simulink model "VCU_TDN"  (R2020a)
settings: Solver=FixedStepDiscrete  StartTime=0.0  StopTime=10.0  FixedStep=0.001  RelTol=1e-3  EnableMultiTasking=on
InitFcn:
  | EcoCoder_PreCheckLic();
undefined symbols (not defined in the file or in its folder): h, km
libraries: CoderSF_BSW_Libs x187, simulink x9, SF_CanService_Libs x1
(part 1 of 2)
settings Model: Creator=timot  LastModifiedBy=Thibault NOUVELLON
settings DataIOCC: SaveFormat=Structure  SignalLoggingSaveFormat=ModelDataLogs  SaveOutput=off  SignalLogging=off  DSMLogging=off  SaveTime=off  ReturnWorkspaceOutputs=off
settings OptimizationCC: DefaultParameterBehavior=Inlined  InlineInvariantSignals=on  EnhancedBackFolding=on  StrengthReduction=on  EnableMemcpy=off  PassReuseOutputArgsAs=Individual arguments  EfficientFloat2IntCast=on  LifeSpan=1  SimCompilerOptimization=on  OptimizeBlockOrder=speed  DifferentSizesBufferReuse=on  EfficientTunableParamExpr=on
settings DebuggingCC: AlgebraicLoopMsg=none  ArtificialAlgebraicLoopMsg=none  SaveWithDisabledLinksMsg=none  SaveWithParameterizedLinksMsg=none  CheckSSInitialOutputMsg=off  UnderspecifiedInitializationDetection=Classic  SignalResolutionControl=TryResolveAll  BlockPriorityViolationMsg=error  MinStepSizeMsg=none  InheritedTsInSrcMsg=none  MultiTaskDSMMsg=none  MultiTaskCondExecSysMsg=none  MultiTaskRateTransMsg=warning  TasksWithSamePriorityMsg=none  SigSpecEnsureSampleTimeMsg=none  IntegerOverflowMsg=error  Int32ToFloatConvMsg=none  ParameterPrecisionLossMsg=none  ParameterTunabilityLossMsg=none  FixptConstOverflowMsg=error  FcnCallInpInsideContextMsg=warning  UnconnectedInputMsg=error  UnconnectedOutputMsg=error  UnconnectedLineMsg=error  FrameProcessingCompatibilityMsg=none  BusObjectLabelMismatch=none  RootOutportRequireBusObject=none  UnknownTsInhSupMsg=none  ModelReferenceDataLoggingMessage=none  OperatingPointInterfaceChecksumMismatchMsg=none  SFUnusedDataAndEventsDiag=none  SFUnexpectedBacktrackingDiag=none  SFInvalidInputDataAccessInChartInitDiag=none  SFNoUnconditionalDefaultTransitionDiag=none  SFTransitionOutsideNaturalParentDiag=none  SFUnreachableExecutionPathDiag=none  SFMachineParentedDataDiag=error
settings HardwareCC: ProdBitPerPointer=32  ProdBitPerSizeT=32  ProdBitPerPtrDiffT=32  ProdLargestAtomicInteger=Long  ProdLargestAtomicFloat=Double  ProdEndianess=BigEndian  ProdWordSize=32  ProdHWDeviceType=Freescale->MPC55xx
settings ModelReferenceCC: UpdateModelReferenceTargets=Force  ModelReferenceNumInstancesAllowed=Single  PropagateSignalLabelsOutOfModel=off
settings SFSimCC: SFSimEcho=off  MATLABDynamicMemAlloc=off
settings RTWCC: Description=Ecotrons MPC5xxx  SystemTargetFile=MPC5644A.tlc  GenerateMakefile=off  TemplateMakefile=ert_default_tmf  RTWVerbose=off  RetainRTWFile=on  RTWCompilerOptimization=on
settings CodeAppCC: IgnoreCustomStorageClasses=off  OperatorAnnotations=on  CustomSymbolStrGlobalVar=$N$M  CustomSymbolStrType=$N$M  CustomSymbolStrFcn=$N$M  CustomSymbolStrFcnArg=$N$M  CustomSymbolStrBlkIO=$N$M  CustomSymbolStrMacro=$N$M
settings STFCustomTargetCC: UtilityFuncGeneration=Shared location  MultiwordLength=256  IncludeMdlTerminateFcn=off  CombineOutputUpdateFcns=on  SuppressErrorStatus=on  ERTCustomFileBanners=on  SupportNonFinite=off  SupportComplex=off  SupportContinuousTime=off  SupportNonInlinedSFcns=off  MATLABClassNameForMDSCustomization=Simulink.SoftwareTarget.ERTCustomization  SystemTargetFile=MPC5644A.tlc
settings ERTTargetCC: UtilityFuncGeneration=Shared location  ParMdlRefBuildCompliant=off  CompOptLevelCompliant=off  ConcurrentExecutionCompliant=off  IncludeMdlTerminateFcn=off  SuppressErrorStatus=on  SupportNonFinite=off  SupportComplex=off  RemoveResetFunc=off  ModelStepFunctionPrototypeControlCompliant=off  CPPClassGenCompliant=off  UseToolchainInfoCompliant=off  GenerateASAP2=on  InlinedParameterPlacement=NonHierarchical  ERTCustomFileTemplate=MPC5644A_file_process.tlc  ERTFilePackagingFormat=Compact  PreserveIfCondition=on  ConvertIfToSwitch=off  PreserveExternInFcnDecls=off  SuppressUnreachableDefaultCases=off

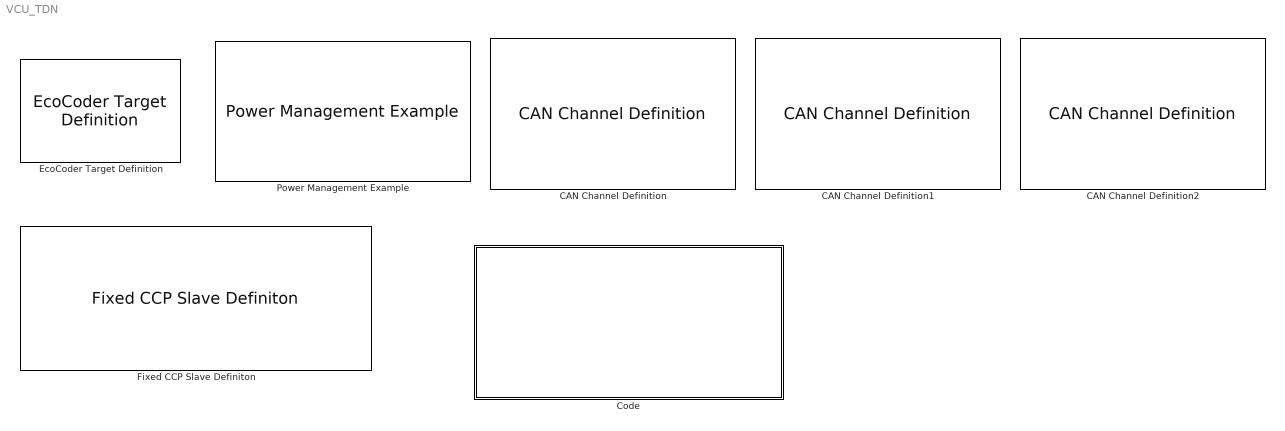
== system VCU_TDN ==
  CAN Channel Definition : CoderSF_BSW_Libs/CAN/CAN Channel Definition  Priority=2  channel=CAN_A  can_en=on  can_idfilter=off  can_rxextended=off  can_rxMask=hex2dec('7ff')  can_rxID=hex2dec('100')  can_baudrateIndex=500  can_txbuffer_size=30  can_rxbuffer_size=1  can_en_fd=off  nominalSamplePoint=7500  can_baudrateIndex_data=500  fastSamplePoint=7500  canfd_txbuffer_size=5  EcoCoderBlockID=C001_CANDef
  CAN Channel Definition1 : CoderSF_BSW_Libs/CAN/CAN Channel Definition  Priority=3  channel=CAN_B  can_en=on  can_idfilter=off  can_rxextended=off  can_rxMask=hex2dec('7ff')  can_rxID=hex2dec('100')  can_baudrateIndex=500  can_txbuffer_size=30  can_rxbuffer_size=1  can_en_fd=off  nominalSamplePoint=7500  can_baudrateIndex_data=500  fastSamplePoint=7500  canfd_txbuffer_size=5  EcoCoderBlockID=C001_CANDef
  CAN Channel Definition2 : CoderSF_BSW_Libs/CAN/CAN Channel Definition  Priority=4  channel=CAN_C  can_en=on  can_idfilter=off  can_rxextended=off  can_rxMask=hex2dec('7ff')  can_rxID=hex2dec('100')  can_baudrateIndex=500  can_txbuffer_size=30  can_rxbuffer_size=1  can_en_fd=off  nominalSamplePoint=7500  can_baudrateIndex_data=500  fastSamplePoint=7500  canfd_txbuffer_size=5  EcoCoderBlockID=C001_CANDef
  Code : Subsystem  Priority=6
  EcoCoder Target Definition : CoderSF_BSW_Libs/EcoCoder Target Definition  targetECU=EV2274A  EcoCoderBlockID=T001_Target  enNoTriggerCall=on  flgBlockReduction=on  flgShowDebugDisp=off  flgDisTargetOutFIleCounter=off  flgClearAllOldFiles=on  tc275_cal_len=hex2dec('00008000')  internal_flash=[hex2dec('00020000'),hex2dec('000E0000')]  cal_rom_phy=[hex2dec('00010000'),hex2dec('00002000')]  cal_ram_wp=[hex2dec('4000F000'),hex2dec('00002000')]  cal_ram_msm=[hex2dec('40000000'),hex2dec('00002000')]  var_ram_wp=[hex2dec('40002000'),hex2dec('0000D000')]  write_back_fixed_ram=[hex2dec('40011000'),hex2dec('00001000')]  write_back_unfixed_ram=[hex2dec('40012000'),hex2dec('00001000')]  stack=[hex2dec('40013000'),hex2dec('00001000')]
      settings: AttributesFormatString=Target :%<targetECU>
  Fixed CCP Slave Definiton : CoderSF_BSW_Libs/CCP/Fixed CCP Slave Definiton  Priority=5  ccpType=Configurable  ccp_enSet=on  ccp_disASW=on  channel=CAN_B  stationaddressSet=hex2dec('0112')  croidSet=hex2dec('100')  dtoidSet=hex2dec('101')  daqidSet=[hex2dec('101') hex2dec('101') hex2dec('101') hex2dec('102')]  daqpidSet=[hex2dec('0') hex2dec('3C') hex2dec('78') hex2dec('0')]  daqlenSet=[hex2dec('0') hex2dec('20') hex2dec('30') hex2dec('30')]  daqperSet=[5 20 100 0]  EcoCoderBlockID=C002_CCP21Conf
  Power Management Example : CoderSF_BSW_Libs/System Management Blocks/Power Management Example  Priority=1  flgKeyFromIn=off  tKeyOffDelaySet=0.5  flgResetSWEnSet=1  tDbncKeyOffFallSet=0.1  tDbncKeyOffRiseSet=0.1  facAd2VoltSet=109/27846  uKeyOffThrSet=1  uKeyOnHystSet=1  flgCANRxLiveCheckEn=0  flgEnPwrDwnFailReset=0  flgNVMEn=on  tShtDwnWait=500  flgPwrDwnByEdgeTrigger=off  EcoCoderBlockID=PME001_Def
      settings: AttributesFormatString=Priority:%<Priority>

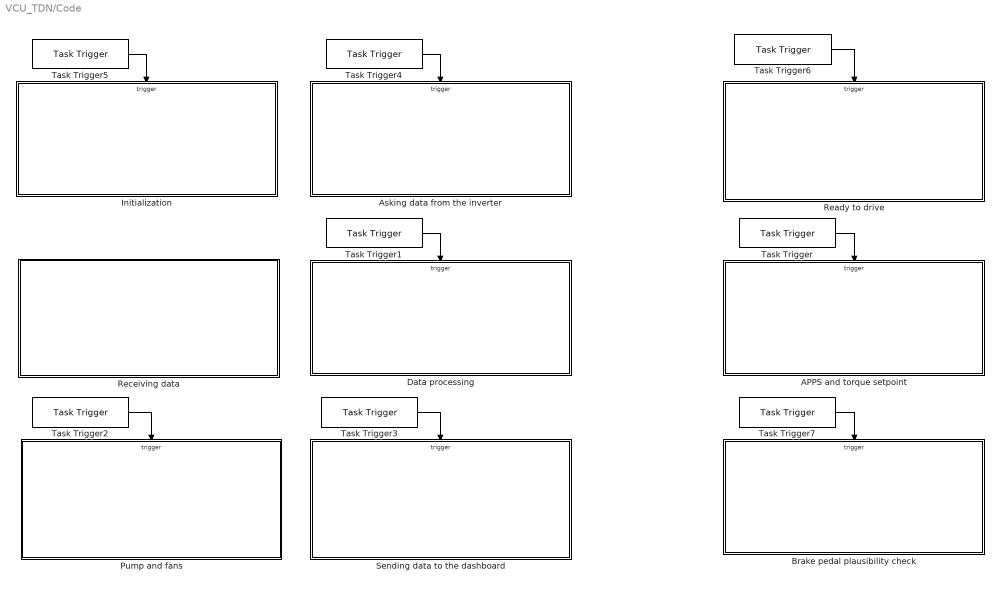
== system VCU_TDN/Code ==
  APPS and torque setpoint : Subsystem
  Asking data from the inverter : Subsystem
  Brake pedal plausibility check : Subsystem
  Data processing : Subsystem
  Initialization : Subsystem
  Pump and fans : Subsystem
  Ready to drive : Subsystem
  Receiving data : Subsystem
  Sending data to the dashboard : Subsystem
  Task Trigger : CoderSF_BSW_Libs/Task Scheduler/Task Trigger  Priority=1  tasktimeIndex=Task_H1ms  PrioritySet=1
  Task Trigger1 : CoderSF_BSW_Libs/Task Scheduler/Task Trigger  Priority=1  tasktimeIndex=Task_L100ms  PrioritySet=1
  Task Trigger2 : CoderSF_BSW_Libs/Task Scheduler/Task Trigger  Priority=1  tasktimeIndex=Task_L1000ms  PrioritySet=1
  Task Trigger3 : CoderSF_BSW_Libs/Task Scheduler/Task Trigger  Priority=2  tasktimeIndex=Task_L100ms  PrioritySet=2
  Task Trigger4 : CoderSF_BSW_Libs/Task Scheduler/Task Trigger  Priority=2  tasktimeIndex=Task_ini  PrioritySet=2
  Task Trigger5 : CoderSF_BSW_Libs/Task Scheduler/Task Trigger  Priority=1  tasktimeIndex=Task_ini  PrioritySet=1
  Task Trigger6 : CoderSF_BSW_Libs/Task Scheduler/Task Trigger  Priority=3  tasktimeIndex=Task_H1ms  PrioritySet=3
  Task Trigger7 : CoderSF_BSW_Libs/Task Scheduler/Task Trigger  Priority=2  tasktimeIndex=Task_H1ms  PrioritySet=2
  wires:
  Task Trigger/1 -> APPS and torque setpoint/Trigger
  Task Trigger3/1 -> Sending data to the dashboard/Trigger
  Task Trigger4/1 -> Asking data from the inverter/Trigger
  Task Trigger1/1 -> Data processing/Trigger
  Task Trigger2/1 -> Pump and fans/Trigger
  Task Trigger5/1 -> Initialization/Trigger
  Task Trigger6/1 -> Ready to drive/Trigger
  Task Trigger7/1 -> Brake pedal plausibility check/Trigger

== system VCU_TDN/Code/APPS and torque setpoint ==
  Trigger : TriggerPort  TriggerType=function-call  VariantControl=Variant  PortDimensions=1
  APPS 1 : CoderSF_BSW_Libs/ADC/Read ADC Value  channel=6
  APPS 2 : CoderSF_BSW_Libs/ADC/Read ADC Value  channel=7
  APPS Fault detection : Subsystem
  Throttle setpoint for the inverter : Subsystem
  Write NVM : CoderSF_BSW_Libs/Non-volatile Memory Blocks/Write NVM  variable_name=nvmAPPS_1  flgDef=on  variable_value=0  variable_type=uint16  variable_numD=1  unitStr=""  descStr=""  EcoCoderBlockID=N001_NVMVDEF
      settings: AttributesFormatString=value:%<variable_value> type:%<variable_type> D:%<variable_numD>
  Write NVM1 : CoderSF_BSW_Libs/Non-volatile Memory Blocks/Write NVM  variable_name=nvmAPPS_2  flgDef=on  variable_value=0  variable_type=uint16  variable_numD=1  unitStr=""  descStr=""  EcoCoderBlockID=N001_NVMVDEF
      settings: AttributesFormatString=value:%<variable_value> type:%<variable_type> D:%<variable_numD>
  Write and Read Measurement : CoderSF_BSW_Libs/Calibration & Measurement/Write and Read Measurement  variable_name=APPS_1  variable_value=0  variable_type=uint16  numD=1  unitStr=""  descStr=""
      settings: AttributesFormatString=type:%<variable_type> Dimensions:%<numD>
  Write and Read Measurement1 : CoderSF_BSW_Libs/Calibration & Measurement/Write and Read Measurement  variable_name=APPS_2  variable_value=0  variable_type=uint16  numD=1  unitStr=""  descStr=""
      settings: AttributesFormatString=type:%<variable_type> Dimensions:%<numD>
  wires:
  APPS 1/1 -> Write NVM/1, Write and Read Measurement/1
  Write and Read Measurement/1 -> Throttle setpoint for the inverter/1(APPS 1), APPS Fault detection/1(APPS 1)  "APPS_1"
  APPS 2/1 -> Write NVM1/1, Write and Read Measurement1/1
  Write and Read Measurement1/1 -> Throttle setpoint for the inverter/2(APPS 2), APPS Fault detection/2(APPS 2)  "APPS_2"

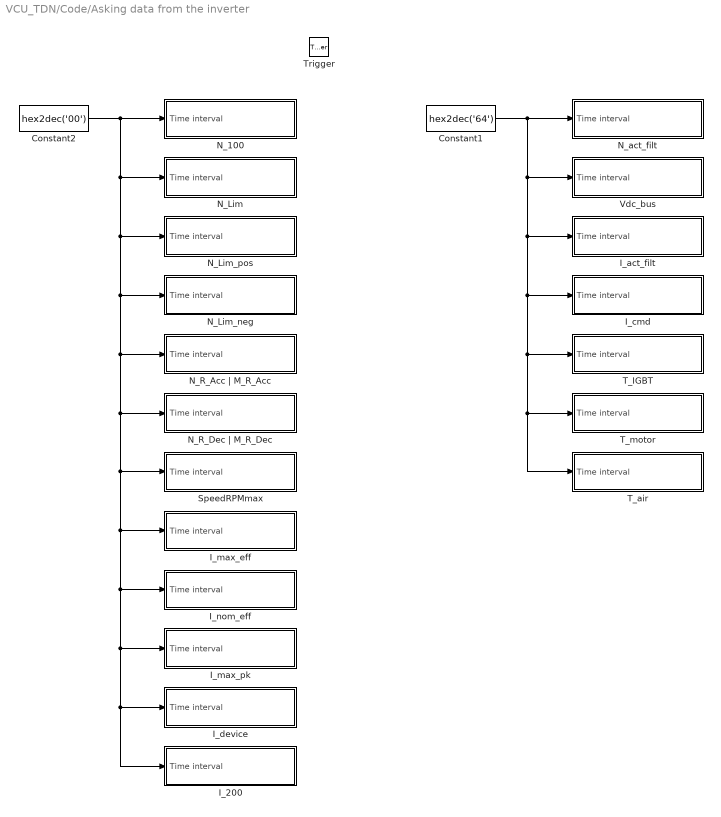
== system VCU_TDN/Code/Asking data from the inverter ==
  Trigger : TriggerPort  TriggerType=function-call  VariantControl=Variant  PortDimensions=1
  Constant1 : Constant  Value=hex2dec('64')  OutDataTypeStr=uint8
  Constant2 : Constant  Value=hex2dec('00')  OutDataTypeStr=uint8
  I_200 : Subsystem
  I_act_filt : Subsystem
  I_cmd : Subsystem
  I_device : Subsystem
  I_max_eff : Subsystem
  I_max_pk : Subsystem
  I_nom_eff : Subsystem
  N_100 : Subsystem
  N_Lim : Subsystem
  N_Lim_neg : Subsystem
  N_Lim_pos : Subsystem
  N_R_Acc | M_R_Acc : Subsystem
  N_R_Dec | M_R_Dec : Subsystem
  N_act_filt : Subsystem
  SpeedRPMmax : Subsystem
  T_IGBT : Subsystem
  T_air : Subsystem
  T_motor : Subsystem
  Vdc_bus : Subsystem
  wires:
  Constant2/1 -> SpeedRPMmax/1(Time interval), I_200/1(Time interval), I_device/1(Time interval), I_max_pk/1(Time interval), I_nom_eff/1(Time interval), I_max_eff/1(Time interval), N_R_Dec | M_R_Dec/1(Time interval), N_R_Acc | M_R_Acc/1(Time interval), N_Lim_neg/1(Time interval), N_Lim_pos/1(Time interval), N_Lim/1(Time interval), N_100/1(Time interval)
  Constant1/1 -> T_air/1(Time interval), T_motor/1(Time interval), T_IGBT/1(Time interval), I_cmd/1(Time interval), I_act_filt/1(Time interval), Vdc_bus/1(Time interval), N_act_filt/1(Time interval)

== system VCU_TDN/Code/Brake pedal plausibility check ==
  Trigger : TriggerPort  TriggerType=function-call  VariantControl=Variant  PortDimensions=1
  Compare To Constant : simulink/Logic and Bit Operations/Compare To Constant  relop=>=  const=5  OutDataTypeStr=boolean
  Logical Operator : Logic  AllPortsSameDT=off  OutDataTypeStr=boolean
  Logical Operator1 : Logic  Inputs=1  AllPortsSameDT=off  OutDataTypeStr=boolean
  Read NVM : CoderSF_BSW_Libs/Non-volatile Memory Blocks/Read NVM  variable_name=nvmAPPS_M  variable_type=Inherit from 'Variable definition'
  Read NVM1 : CoderSF_BSW_Libs/Non-volatile Memory Blocks/Read NVM  variable_name=nvmBRK_CONTACTOR  variable_type=Inherit from 'Variable definition'
  Tapped Delay : simulink/Discrete/Tapped Delay  vinit=0.0  samptime=-1  NumDelays=490  DelayOrder=Oldest  includeCurrent=off
  Write Measurement : CoderSF_BSW_Libs/Calibration & Measurement/Write Measurement  variable_name=BRK_PDL_FAULT  variable_value=0  variable_type=boolean  numD=1  unitStr=""  descStr=""
      settings: AttributesFormatString=type:%<variable_type> Dimensions:%<numD>
  Write NVM : CoderSF_BSW_Libs/Non-volatile Memory Blocks/Write NVM  variable_name=nvmBRK_PDL_FAULT  flgDef=on  variable_value=0  variable_type=boolean  variable_numD=1  unitStr=""  descStr=""  EcoCoderBlockID=N001_NVMVDEF
      settings: AttributesFormatString=value:%<variable_value> type:%<variable_type> D:%<variable_numD>
  wires:
  Read NVM1/1 -> Logical Operator/2
  Logical Operator/1 -> Tapped Delay/1
  Tapped Delay/1 -> Logical Operator1/1
  Read NVM/1 -> Compare To Constant/1
  Compare To Constant/1 -> Logical Operator/1
  Logical Operator1/1 -> Write NVM/1, Write Measurement/1

== system VCU_TDN/Code/Data processing ==
  Trigger : TriggerPort  TriggerType=function-call  VariantControl=Variant  PortDimensions=1
  Electrical : Subsystem
  Speed : Subsystem
  Temperature : Subsystem

== system VCU_TDN/Code/Initialization ==
  Trigger : TriggerPort  TriggerType=function-call  VariantControl=Variant  PortDimensions=1
  Constant : Constant  Value=0  OutDataTypeStr=boolean
  Constant1 : Constant  Value=0  OutDataTypeStr=boolean
  Disabling the inverter : Subsystem
  FRG/RUN : CoderSF_BSW_Libs/Digital I//O/Switch Output  channel=LSO07
  NVM Definition : CoderSF_BSW_Libs/Non-volatile Memory Blocks/NVM Definition  load=Restore from factory default values in .mot  EcoCoderBlockID=N001_NVMDef
  RFE : CoderSF_BSW_Libs/Digital I//O/Switch Output  channel=LSO06
  wires:
  Constant/1 -> RFE/1
  Constant1/1 -> FRG/RUN/1

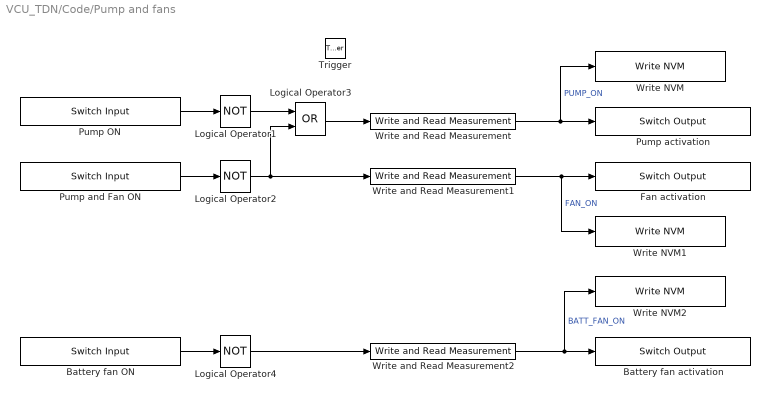
== system VCU_TDN/Code/Pump and fans ==
  Trigger : TriggerPort  TriggerType=function-call  VariantControl=Variant  PortDimensions=1
  Battery fan ON : CoderSF_BSW_Libs/Digital I//O/Switch Input  portNum=DI09
  Battery fan activation : CoderSF_BSW_Libs/Digital I//O/Switch Output  channel=LSO03
  Fan activation : CoderSF_BSW_Libs/Digital I//O/Switch Output  channel=LSO13
  Logical Operator1 : Logic  Operator=NOT  AllPortsSameDT=off  OutDataTypeStr=boolean
  Logical Operator2 : Logic  Operator=NOT  AllPortsSameDT=off  OutDataTypeStr=boolean
  Logical Operator3 : Logic  Operator=OR  AllPortsSameDT=off  OutDataTypeStr=boolean
  Logical Operator4 : Logic  Operator=NOT  AllPortsSameDT=off  OutDataTypeStr=boolean
  Pump ON : CoderSF_BSW_Libs/Digital I//O/Switch Input  portNum=DI12
  Pump activation : CoderSF_BSW_Libs/Digital I//O/Switch Output  channel=LSO12
  Pump and Fan ON : CoderSF_BSW_Libs/Digital I//O/Switch Input  portNum=DI12
  Write NVM : CoderSF_BSW_Libs/Non-volatile Memory Blocks/Write NVM  variable_name=nvmPUMP_ON  flgDef=on  variable_value=0  variable_type=boolean  variable_numD=1  unitStr=""  descStr=""  EcoCoderBlockID=N001_NVMVDEF
      settings: AttributesFormatString=value:%<variable_value> type:%<variable_type> D:%<variable_numD>
  Write NVM1 : CoderSF_BSW_Libs/Non-volatile Memory Blocks/Write NVM  variable_name=nvmFAN_ON  flgDef=on  variable_value=0  variable_type=boolean  variable_numD=1  unitStr=""  descStr=""  EcoCoderBlockID=N001_NVMVDEF
      settings: AttributesFormatString=value:%<variable_value> type:%<variable_type> D:%<variable_numD>
  Write NVM2 : CoderSF_BSW_Libs/Non-volatile Memory Blocks/Write NVM  variable_name=nvmBATT_FAN_ON  flgDef=on  variable_value=0  variable_type=boolean  variable_numD=1  unitStr=""  descStr=""  EcoCoderBlockID=N001_NVMVDEF
      settings: AttributesFormatString=value:%<variable_value> type:%<variable_type> D:%<variable_numD>
  Write and Read Measurement : CoderSF_BSW_Libs/Calibration & Measurement/Write and Read Measurement  variable_name=PUMP_ON  variable_value=0  variable_type=boolean  numD=1  unitStr=""  descStr=""
      settings: AttributesFormatString=type:%<variable_type> Dimensions:%<numD>
  Write and Read Measurement1 : CoderSF_BSW_Libs/Calibration & Measurement/Write and Read Measurement  variable_name=FAN_ON  variable_value=0  variable_type=boolean  numD=1  unitStr=""  descStr=""
      settings: AttributesFormatString=type:%<variable_type> Dimensions:%<numD>
  Write and Read Measurement2 : CoderSF_BSW_Libs/Calibration & Measurement/Write and Read Measurement  variable_name=BATT_FAN_ON  variable_value=0  variable_type=boolean  numD=1  unitStr=""  descStr=""
      settings: AttributesFormatString=type:%<variable_type> Dimensions:%<numD>
  wires:
  Logical Operator2/1 -> Write and Read Measurement1/1, Logical Operator3/2
  Pump and Fan ON/1 -> Logical Operator2/1
  Logical Operator1/1 -> Logical Operator3/1
  Logical Operator4/1 -> Write and Read Measurement2/1
  Logical Operator3/1 -> Write and Read Measurement/1
  Battery fan ON/1 -> Logical Operator4/1
  Pump ON/1 -> Logical Operator1/1
  Write and Read Measurement2/1 -> Write NVM2/1, Battery fan activation/1  "BATT_FAN_ON"
  Write and Read Measurement1/1 -> Write NVM1/1, Fan activation/1  "FAN_ON"
  Write and Read Measurement/1 -> Write NVM/1, Pump activation/1  "PUMP_ON"

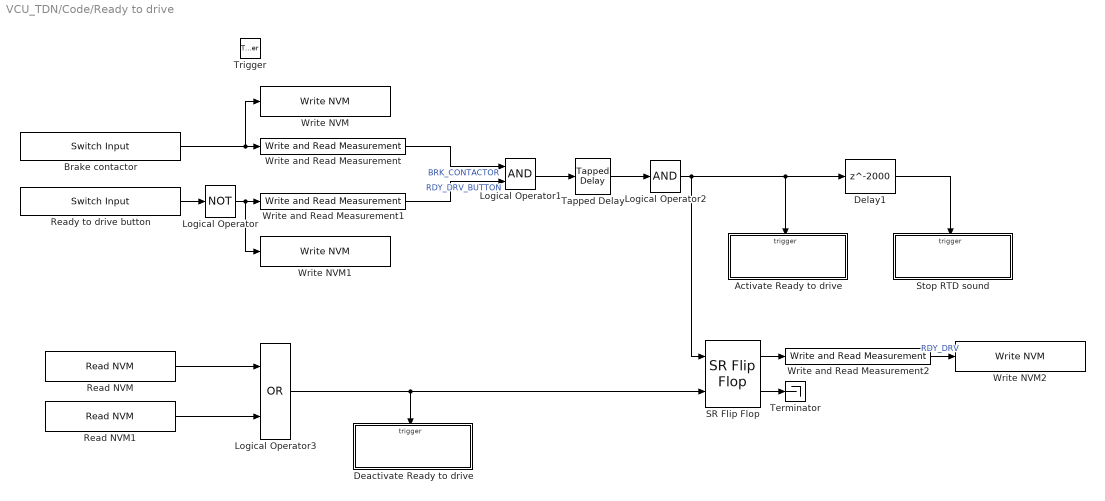
== system VCU_TDN/Code/Ready to drive ==
  Trigger : TriggerPort  TriggerType=function-call  VariantControl=Variant  PortDimensions=1
  Activate Ready to drive : Subsystem  TreatAsAtomicUnit=on
  Brake contactor : CoderSF_BSW_Libs/Digital I//O/Switch Input  portNum=DI18
  Deactivate Ready to drive : Subsystem  TreatAsAtomicUnit=on
  Delay1 : Delay  DelayLength=2000
  Logical Operator : Logic  Operator=NOT  AllPortsSameDT=off  OutDataTypeStr=boolean
  Logical Operator1 : Logic  AllPortsSameDT=off  OutDataTypeStr=boolean
  Logical Operator2 : Logic  Inputs=1  AllPortsSameDT=off  OutDataTypeStr=boolean
  Logical Operator3 : Logic  Operator=OR  AllPortsSameDT=off  OutDataTypeStr=boolean
  Read NVM : CoderSF_BSW_Libs/Non-volatile Memory Blocks/Read NVM  variable_name=nvmAPPS_FAULT  variable_type=Inherit from 'Variable definition'
  Read NVM1 : CoderSF_BSW_Libs/Non-volatile Memory Blocks/Read NVM  variable_name=nvmBRK_PDL_FAULT  variable_type=Inherit from 'Variable definition'
  Ready to drive button : CoderSF_BSW_Libs/Digital I//O/Switch Input  portNum=DI01
  SR Flip Flop : CoderSF_BSW_Libs/Application Base Blocks/SR Flip Flop
  Stop RTD sound : Subsystem  TreatAsAtomicUnit=on
  Tapped Delay : simulink/Discrete/Tapped Delay  vinit=0.0  samptime=-1  NumDelays=1000  DelayOrder=Oldest  includeCurrent=off
  Terminator : Terminator
  Write NVM : CoderSF_BSW_Libs/Non-volatile Memory Blocks/Write NVM  variable_name=nvmBRK_CONTACTOR  flgDef=on  variable_value=0  variable_type=boolean  variable_numD=1  unitStr=""  descStr=""  EcoCoderBlockID=N001_NVMVDEF
      settings: AttributesFormatString=value:%<variable_value> type:%<variable_type> D:%<variable_numD>
  Write NVM1 : CoderSF_BSW_Libs/Non-volatile Memory Blocks/Write NVM  variable_name=nvmRDY_DRV_BUTTON  flgDef=on  variable_value=0  variable_type=boolean  variable_numD=1  unitStr=""  descStr=""  EcoCoderBlockID=N001_NVMVDEF
      settings: AttributesFormatString=value:%<variable_value> type:%<variable_type> D:%<variable_numD>
  Write NVM2 : CoderSF_BSW_Libs/Non-volatile Memory Blocks/Write NVM  variable_name=nvmRDY_DRV  flgDef=on  variable_value=0  variable_type=boolean  variable_numD=1  unitStr=""  descStr=""  EcoCoderBlockID=N001_NVMVDEF
      settings: AttributesFormatString=value:%<variable_value> type:%<variable_type> D:%<variable_numD>
  Write and Read Measurement : CoderSF_BSW_Libs/Calibration & Measurement/Write and Read Measurement  variable_name=BRK_CONTACTOR  variable_value=0  variable_type=boolean  numD=1  unitStr=""  descStr=""
      settings: AttributesFormatString=type:%<variable_type> Dimensions:%<numD>
  Write and Read Measurement1 : CoderSF_BSW_Libs/Calibration & Measurement/Write and Read Measurement  variable_name=RDY_DRV_BUTTON  variable_value=0  variable_type=boolean  numD=1  unitStr=""  descStr=""
      settings: AttributesFormatString=type:%<variable_type> Dimensions:%<numD>
  Write and Read Measurement2 : CoderSF_BSW_Libs/Calibration & Measurement/Write and Read Measurement  variable_name=RDY_DRV  variable_value=0  variable_type=boolean  numD=1  unitStr=""  descStr=""
      settings: AttributesFormatString=type:%<variable_type> Dimensions:%<numD>
  wires:
  Ready to drive button/1 -> Logical Operator/1
  Brake contactor/1 -> Write NVM/1, Write and Read Measurement/1
  Logical Operator/1 -> Write NVM1/1, Write and Read Measurement1/1
  Write and Read Measurement/1 -> Logical Operator1/1  "BRK_CONTACTOR"
  Write and Read Measurement1/1 -> Logical Operator1/2  "RDY_DRV_BUTTON"
  Logical Operator1/1 -> Tapped Delay/1
  Read NVM/1 -> Logical Operator3/1
  Logical Operator3/1 -> Deactivate Ready to drive/Trigger, SR Flip Flop/2
  Read NVM1/1 -> Logical Operator3/2
  Logical Operator2/1 -> Delay1/1, Activate Ready to drive/Trigger, SR Flip Flop/1
  Tapped Delay/1 -> Logical Operator2/1
  Delay1/1 -> Stop RTD sound/Trigger
  SR Flip Flop/1 -> Write and Read Measurement2/1
  Write and Read Measurement2/1 -> Write NVM2/1  "RDY_DRV"
  SR Flip Flop/2 -> Terminator/1

== system VCU_TDN/Code/Receiving data ==
  BMS : Subsystem
  Battery temperature sensors : Subsystem
  Inverter : Subsystem
  Sensors : Subsystem
  Task Trigger1 : CoderSF_BSW_Libs/Task Scheduler/Task Trigger  Priority=3  tasktimeIndex=Task_L100ms  PrioritySet=3
  wires:
  Task Trigger1/1 -> Sensors/Trigger

== system VCU_TDN/Code/Sending data to the dashboard ==
  Trigger : TriggerPort  TriggerType=function-call  VariantControl=Variant  PortDimensions=1
  Read NVM : CoderSF_BSW_Libs/Non-volatile Memory Blocks/Read NVM  variable_name=nvmSpeed  variable_type=Inherit from 'Variable definition'
  Terminator : Terminator
  wires:
  Read NVM/1 -> Terminator/1

== system VCU_TDN/Code/APPS and torque setpoint/APPS Fault detection ==
  APPS 1 : Inport
  APPS 2 : Inport  Port=2
  Abs : Abs
  Compare To Constant : simulink/Logic and Bit Operations/Compare To Constant  relop=>=  const=0.09*4096  OutDataTypeStr=boolean
  Logical Operator1 : Logic  Inputs=1  AllPortsSameDT=off  OutDataTypeStr=boolean
  Subtract : Sum  Inputs=+-
  Tapped Delay : simulink/Discrete/Tapped Delay  vinit=0.0  samptime=-1  NumDelays=90  DelayOrder=Oldest  includeCurrent=off
  Write Measurement : CoderSF_BSW_Libs/Calibration & Measurement/Write Measurement  variable_name=APPS_FAULT  variable_value=0  variable_type=boolean  numD=1  unitStr=""  descStr=""
      settings: AttributesFormatString=type:%<variable_type> Dimensions:%<numD>
  Write NVM : CoderSF_BSW_Libs/Non-volatile Memory Blocks/Write NVM  variable_name=nvmAPPS_FAULT  flgDef=on  variable_value=0  variable_type=boolean  variable_numD=1  unitStr=""  descStr=""  EcoCoderBlockID=N001_NVMVDEF
      settings: AttributesFormatString=value:%<variable_value> type:%<variable_type> D:%<variable_numD>
  wires:
  APPS 1/1 -> Subtract/1
  Subtract/1 -> Abs/1
  Compare To Constant/1 -> Tapped Delay/1
  Abs/1 -> Compare To Constant/1
  Logical Operator1/1 -> Write NVM/1, Write Measurement/1
  APPS 2/1 -> Subtract/2
  Tapped Delay/1 -> Logical Operator1/1

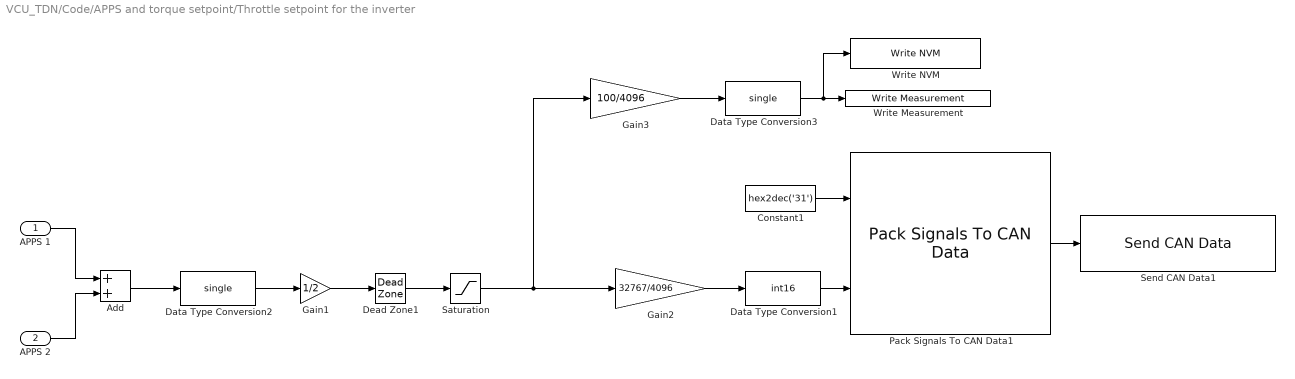
== system VCU_TDN/Code/APPS and torque setpoint/Throttle setpoint for the inverter ==
  APPS 1 : Inport
  APPS 2 : Inport  Port=2
  Add : Sum
  Constant1 : Constant  Value=hex2dec('31')  OutDataTypeStr=uint8
  Data Type Conversion1 : DataTypeConversion  OutDataTypeStr=int16
  Data Type Conversion2 : DataTypeConversion  OutDataTypeStr=single
  Data Type Conversion3 : DataTypeConversion  OutDataTypeStr=single
  Dead Zone1 : DeadZone  LowerValue=-5  UpperValue=5  SaturateOnIntegerOverflow=on
  Gain1 : Gain  Gain=1/2
  Gain2 : Gain  Gain=32767/4096
  Gain3 : Gain  Gain=100/4096
  Pack Signals To CAN Data1 : CoderSF_BSW_Libs/CAN/Pack Signals To CAN Data  Signal="{{'REG_31'  'Data1'},[0 8],[8 16],{'uint8'  'int16'},{'Intel' 'Intel'}}"
  Saturation : Saturate  UpperLimit=4096  LowerLimit=0
  Send CAN Data1 : CoderSF_BSW_Libs/CAN/Send CAN Data  channel=CAN_A  txlen=3  txid=hex2dec('201')  frametype=Standard(11-bit ID)  showerror=off
  Write Measurement : CoderSF_BSW_Libs/Calibration & Measurement/Write Measurement  variable_name=APPS_M  variable_value=0  variable_type=single  numD=1  unitStr=%  descStr=""
      settings: AttributesFormatString=type:%<variable_type> Dimensions:%<numD>
  Write NVM : CoderSF_BSW_Libs/Non-volatile Memory Blocks/Write NVM  variable_name=nvmAPPS_M  flgDef=on  variable_value=0  variable_type=single  variable_numD=1  unitStr=%  descStr=""  EcoCoderBlockID=N001_NVMVDEF
      settings: AttributesFormatString=value:%<variable_value> type:%<variable_type> D:%<variable_numD>
  wires:
  APPS 1/1 -> Add/1
  Gain1/1 -> Dead Zone1/1
  Pack Signals To CAN Data1/1 -> Send CAN Data1/1
  Gain2/1 -> Data Type Conversion1/1
  Data Type Conversion1/1 -> Pack Signals To CAN Data1/2
  Constant1/1 -> Pack Signals To CAN Data1/1
  APPS 2/1 -> Add/2
  Gain3/1 -> Data Type Conversion3/1
  Data Type Conversion3/1 -> Write NVM/1, Write Measurement/1
  Dead Zone1/1 -> Saturation/1
  Saturation/1 -> Gain3/1, Gain2/1
  Data Type Conversion2/1 -> Gain1/1
  Add/1 -> Data Type Conversion2/1

== system VCU_TDN/Code/Asking data from the inverter/I_200 ==
  Time interval : Inport
  Constant : Constant  Value=hex2dec('3d')  OutDataTypeStr=uint8
  Constant1 : Constant  Value=hex2dec('d9')  OutDataTypeStr=uint8
  Pack Signals To CAN Data : CoderSF_BSW_Libs/CAN/Pack Signals To CAN Data  Signal="{{'REG_31'  'Data1' 'Data2'},[0 8 16],[8 8 8],{'uint8'  'uint8' 'uint8'},{'Intel' 'Intel' 'Intel'}}"
  Send CAN Data : CoderSF_BSW_Libs/CAN/Send CAN Data  channel=CAN_A  txlen=3  txid=hex2dec('201')  frametype=Standard(11-bit ID)  showerror=off
  wires:
  Constant/1 -> Pack Signals To CAN Data/1
  Pack Signals To CAN Data/1 -> Send CAN Data/1
  Constant1/1 -> Pack Signals To CAN Data/2
  Time interval/1 -> Pack Signals To CAN Data/3

== system VCU_TDN/Code/Asking data from the inverter/I_act_filt ==
  Time interval : Inport
  Constant : Constant  Value=hex2dec('3d')  OutDataTypeStr=uint8
  Constant1 : Constant  Value=hex2dec('5f')  OutDataTypeStr=uint8
  Pack Signals To CAN Data : CoderSF_BSW_Libs/CAN/Pack Signals To CAN Data  Signal="{{'REG_31'  'Data1' 'Data2'},[0 8 16],[8 8 8],{'uint8'  'uint8' 'uint8'},{'Intel' 'Intel' 'Intel'}}"
  Send CAN Data : CoderSF_BSW_Libs/CAN/Send CAN Data  channel=CAN_A  txlen=3  txid=hex2dec('201')  frametype=Standard(11-bit ID)  showerror=off
  wires:
  Constant/1 -> Pack Signals To CAN Data/1
  Pack Signals To CAN Data/1 -> Send CAN Data/1
  Constant1/1 -> Pack Signals To CAN Data/2
  Time interval/1 -> Pack Signals To CAN Data/3

== system VCU_TDN/Code/Asking data from the inverter/I_cmd ==
  Time interval : Inport
  Constant : Constant  Value=hex2dec('3d')  OutDataTypeStr=uint8
  Constant1 : Constant  Value=hex2dec('26')  OutDataTypeStr=uint8
  Pack Signals To CAN Data : CoderSF_BSW_Libs/CAN/Pack Signals To CAN Data  Signal="{{'REG_31'  'Data1' 'Data2'},[0 8 16],[8 8 8],{'uint8'  'uint8' 'uint8'},{'Intel' 'Intel' 'Intel'}}"
  Send CAN Data : CoderSF_BSW_Libs/CAN/Send CAN Data  channel=CAN_A  txlen=3  txid=hex2dec('201')  frametype=Standard(11-bit ID)  showerror=off
  wires:
  Constant/1 -> Pack Signals To CAN Data/1
  Pack Signals To CAN Data/1 -> Send CAN Data/1
  Constant1/1 -> Pack Signals To CAN Data/2
  Time interval/1 -> Pack Signals To CAN Data/3

== system VCU_TDN/Code/Asking data from the inverter/I_device ==
  Time interval : Inport
  Constant : Constant  Value=hex2dec('3d')  OutDataTypeStr=uint8
  Constant1 : Constant  Value=hex2dec('c6')  OutDataTypeStr=uint8
  Pack Signals To CAN Data : CoderSF_BSW_Libs/CAN/Pack Signals To CAN Data  Signal="{{'REG_31'  'Data1' 'Data2'},[0 8 16],[8 8 8],{'uint8'  'uint8' 'uint8'},{'Intel' 'Intel' 'Intel'}}"
  Send CAN Data : CoderSF_BSW_Libs/CAN/Send CAN Data  channel=CAN_A  txlen=3  txid=hex2dec('201')  frametype=Standard(11-bit ID)  showerror=off
  wires:
  Constant/1 -> Pack Signals To CAN Data/1
  Pack Signals To CAN Data/1 -> Send CAN Data/1
  Constant1/1 -> Pack Signals To CAN Data/2
  Time interval/1 -> Pack Signals To CAN Data/3

== system VCU_TDN/Code/Asking data from the inverter/I_max_eff ==
  Time interval : Inport
  Constant : Constant  Value=hex2dec('3d')  OutDataTypeStr=uint8
  Constant1 : Constant  Value=hex2dec('4d')  OutDataTypeStr=uint8
  Pack Signals To CAN Data : CoderSF_BSW_Libs/CAN/Pack Signals To CAN Data  Signal="{{'REG_31'  'Data1' 'Data2'},[0 8 16],[8 8 8],{'uint8'  'uint8' 'uint8'},{'Intel' 'Intel' 'Intel'}}"
  Send CAN Data : CoderSF_BSW_Libs/CAN/Send CAN Data  channel=CAN_A  txlen=3  txid=hex2dec('201')  frametype=Standard(11-bit ID)  showerror=off
  wires:
  Constant/1 -> Pack Signals To CAN Data/1
  Pack Signals To CAN Data/1 -> Send CAN Data/1
  Constant1/1 -> Pack Signals To CAN Data/2
  Time interval/1 -> Pack Signals To CAN Data/3

== system VCU_TDN/Code/Asking data from the inverter/I_max_pk ==
  Time interval : Inport
  Constant : Constant  Value=hex2dec('3d')  OutDataTypeStr=uint8
  Constant1 : Constant  Value=hex2dec('c4')  OutDataTypeStr=uint8
  Pack Signals To CAN Data : CoderSF_BSW_Libs/CAN/Pack Signals To CAN Data  Signal="{{'REG_31'  'Data1' 'Data2'},[0 8 16],[8 8 8],{'uint8'  'uint8' 'uint8'},{'Intel' 'Intel' 'Intel'}}"
  Send CAN Data : CoderSF_BSW_Libs/CAN/Send CAN Data  channel=CAN_A  txlen=3  txid=hex2dec('201')  frametype=Standard(11-bit ID)  showerror=off
  wires:
  Constant/1 -> Pack Signals To CAN Data/1
  Pack Signals To CAN Data/1 -> Send CAN Data/1
  Constant1/1 -> Pack Signals To CAN Data/2
  Time interval/1 -> Pack Signals To CAN Data/3

== system VCU_TDN/Code/Asking data from the inverter/I_nom_eff ==
  Time interval : Inport
  Constant : Constant  Value=hex2dec('3d')  OutDataTypeStr=uint8
  Constant1 : Constant  Value=hex2dec('4e')  OutDataTypeStr=uint8
  Pack Signals To CAN Data : CoderSF_BSW_Libs/CAN/Pack Signals To CAN Data  Signal="{{'REG_31'  'Data1' 'Data2'},[0 8 16],[8 8 8],{'uint8'  'uint8' 'uint8'},{'Intel' 'Intel' 'Intel'}}"
  Send CAN Data : CoderSF_BSW_Libs/CAN/Send CAN Data  channel=CAN_A  txlen=3  txid=hex2dec('201')  frametype=Standard(11-bit ID)  showerror=off
  wires:
  Constant/1 -> Pack Signals To CAN Data/1
  Pack Signals To CAN Data/1 -> Send CAN Data/1
  Constant1/1 -> Pack Signals To CAN Data/2
  Time interval/1 -> Pack Signals To CAN Data/3

== system VCU_TDN/Code/Asking data from the inverter/N_100 ==
  Time interval : Inport
  Constant : Constant  Value=hex2dec('3d')  OutDataTypeStr=uint8
  Constant1 : Constant  Value=hex2dec('c8')  OutDataTypeStr=uint8
  Pack Signals To CAN Data : CoderSF_BSW_Libs/CAN/Pack Signals To CAN Data  Signal="{{'REG_31'  'Data1' 'Data2'},[0 8 16],[8 8 8],{'uint8'  'uint8' 'uint8'},{'Intel' 'Intel' 'Intel'}}"
  Send CAN Data : CoderSF_BSW_Libs/CAN/Send CAN Data  channel=CAN_A  txlen=3  txid=hex2dec('201')  frametype=Standard(11-bit ID)  showerror=off
  wires:
  Constant/1 -> Pack Signals To CAN Data/1
  Pack Signals To CAN Data/1 -> Send CAN Data/1
  Constant1/1 -> Pack Signals To CAN Data/2
  Time interval/1 -> Pack Signals To CAN Data/3

== system VCU_TDN/Code/Asking data from the inverter/N_Lim ==
  Time interval : Inport
  Constant : Constant  Value=hex2dec('3d')  OutDataTypeStr=uint8
  Constant1 : Constant  Value=hex2dec('34')  OutDataTypeStr=uint8
  Pack Signals To CAN Data : CoderSF_BSW_Libs/CAN/Pack Signals To CAN Data  Signal="{{'REG_31'  'Data1' 'Data2'},[0 8 16],[8 8 8],{'uint8'  'uint8' 'uint8'},{'Intel' 'Intel' 'Intel'}}"
  Send CAN Data : CoderSF_BSW_Libs/CAN/Send CAN Data  channel=CAN_A  txlen=3  txid=hex2dec('201')  frametype=Standard(11-bit ID)  showerror=off
  wires:
  Constant/1 -> Pack Signals To CAN Data/1
  Pack Signals To CAN Data/1 -> Send CAN Data/1
  Constant1/1 -> Pack Signals To CAN Data/2
  Time interval/1 -> Pack Signals To CAN Data/3

== system VCU_TDN/Code/Asking data from the inverter/N_Lim_neg ==
  Time interval : Inport
  Constant : Constant  Value=hex2dec('3d')  OutDataTypeStr=uint8
  Constant1 : Constant  Value=hex2dec('3e')  OutDataTypeStr=uint8
  Pack Signals To CAN Data : CoderSF_BSW_Libs/CAN/Pack Signals To CAN Data  Signal="{{'REG_31'  'Data1' 'Data2'},[0 8 16],[8 8 8],{'uint8'  'uint8' 'uint8'},{'Intel' 'Intel' 'Intel'}}"
  Send CAN Data : CoderSF_BSW_Libs/CAN/Send CAN Data  channel=CAN_A  txlen=3  txid=hex2dec('201')  frametype=Standard(11-bit ID)  showerror=off
  wires:
  Constant/1 -> Pack Signals To CAN Data/1
  Pack Signals To CAN Data/1 -> Send CAN Data/1
  Constant1/1 -> Pack Signals To CAN Data/2
  Time interval/1 -> Pack Signals To CAN Data/3

== system VCU_TDN/Code/Asking data from the inverter/N_Lim_pos ==
  Time interval : Inport
  Constant : Constant  Value=hex2dec('3d')  OutDataTypeStr=uint8
  Constant1 : Constant  Value=hex2dec('3f')  OutDataTypeStr=uint8
  Pack Signals To CAN Data : CoderSF_BSW_Libs/CAN/Pack Signals To CAN Data  Signal="{{'REG_31'  'Data1' 'Data2'},[0 8 16],[8 8 8],{'uint8'  'uint8' 'uint8'},{'Intel' 'Intel' 'Intel'}}"
  Send CAN Data : CoderSF_BSW_Libs/CAN/Send CAN Data  channel=CAN_A  txlen=3  txid=hex2dec('201')  frametype=Standard(11-bit ID)  showerror=off
  wires:
  Constant/1 -> Pack Signals To CAN Data/1
  Pack Signals To CAN Data/1 -> Send CAN Data/1
  Constant1/1 -> Pack Signals To CAN Data/2
  Time interval/1 -> Pack Signals To CAN Data/3

== system VCU_TDN/Code/Asking data from the inverter/N_R_Acc | M_R_Acc ==
  Time interval : Inport
  Constant : Constant  Value=hex2dec('3d')  OutDataTypeStr=uint8
  Constant1 : Constant  Value=hex2dec('35')  OutDataTypeStr=uint8
  Pack Signals To CAN Data : CoderSF_BSW_Libs/CAN/Pack Signals To CAN Data  Signal="{{'REG_31'  'Data1' 'Data2'},[0 8 16],[8 8 8],{'uint8'  'uint8' 'uint8'},{'Intel' 'Intel' 'Intel'}}"
  Send CAN Data : CoderSF_BSW_Libs/CAN/Send CAN Data  channel=CAN_A  txlen=3  txid=hex2dec('201')  frametype=Standard(11-bit ID)  showerror=off
  wires:
  Constant/1 -> Pack Signals To CAN Data/1
  Pack Signals To CAN Data/1 -> Send CAN Data/1
  Constant1/1 -> Pack Signals To CAN Data/2
  Time interval/1 -> Pack Signals To CAN Data/3

== system VCU_TDN/Code/Asking data from the inverter/N_R_Dec | M_R_Dec ==
  Time interval : Inport
  Constant : Constant  Value=hex2dec('3d')  OutDataTypeStr=uint8
  Constant1 : Constant  Value=hex2dec('ed')  OutDataTypeStr=uint8
  Pack Signals To CAN Data : CoderSF_BSW_Libs/CAN/Pack Signals To CAN Data  Signal="{{'REG_31'  'Data1' 'Data2'},[0 8 16],[8 8 8],{'uint8'  'uint8' 'uint8'},{'Intel' 'Intel' 'Intel'}}"
  Send CAN Data : CoderSF_BSW_Libs/CAN/Send CAN Data  channel=CAN_A  txlen=3  txid=hex2dec('201')  frametype=Standard(11-bit ID)  showerror=off
  wires:
  Constant/1 -> Pack Signals To CAN Data/1
  Pack Signals To CAN Data/1 -> Send CAN Data/1
  Constant1/1 -> Pack Signals To CAN Data/2
  Time interval/1 -> Pack Signals To CAN Data/3

== system VCU_TDN/Code/Asking data from the inverter/N_act_filt ==
  Time interval : Inport
  Constant : Constant  Value=hex2dec('3d')  OutDataTypeStr=uint8
  Constant1 : Constant  Value=hex2dec('a8')  OutDataTypeStr=uint8
  Pack Signals To CAN Data : CoderSF_BSW_Libs/CAN/Pack Signals To CAN Data  Signal="{{'REG_31'  'Data1' 'Data2'},[0 8 16],[8 8 8],{'uint8'  'uint8' 'uint8'},{'Intel' 'Intel' 'Intel'}}"
  Send CAN Data : CoderSF_BSW_Libs/CAN/Send CAN Data  channel=CAN_A  txlen=3  txid=hex2dec('201')  frametype=Standard(11-bit ID)  showerror=off
  wires:
  Constant/1 -> Pack Signals To CAN Data/1
  Pack Signals To CAN Data/1 -> Send CAN Data/1
  Constant1/1 -> Pack Signals To CAN Data/2
  Time interval/1 -> Pack Signals To CAN Data/3

== system VCU_TDN/Code/Asking data from the inverter/SpeedRPMmax ==
  Time interval : Inport
  Constant : Constant  Value=hex2dec('3d')  OutDataTypeStr=uint8
  Constant1 : Constant  Value=hex2dec('ce')  OutDataTypeStr=uint8
  Pack Signals To CAN Data : CoderSF_BSW_Libs/CAN/Pack Signals To CAN Data  Signal="{{'REG_31'  'Data1' 'Data2'},[0 8 16],[8 8 8],{'uint8'  'uint8' 'uint8'},{'Intel' 'Intel' 'Intel'}}"
  Send CAN Data : CoderSF_BSW_Libs/CAN/Send CAN Data  channel=CAN_A  txlen=3  txid=hex2dec('201')  frametype=Standard(11-bit ID)  showerror=off
  wires:
  Constant/1 -> Pack Signals To CAN Data/1
  Pack Signals To CAN Data/1 -> Send CAN Data/1
  Constant1/1 -> Pack Signals To CAN Data/2
  Time interval/1 -> Pack Signals To CAN Data/3

== system VCU_TDN/Code/Asking data from the inverter/T_IGBT ==
  Time interval : Inport
  Constant : Constant  Value=hex2dec('3d')  OutDataTypeStr=uint8
  Constant1 : Constant  Value=hex2dec('4a')  OutDataTypeStr=uint8
  Pack Signals To CAN Data : CoderSF_BSW_Libs/CAN/Pack Signals To CAN Data  Signal="{{'REG_31'  'Data1' 'Data2'},[0 8 16],[8 8 8],{'uint8'  'uint8' 'uint8'},{'Intel' 'Intel' 'Intel'}}"
  Send CAN Data : CoderSF_BSW_Libs/CAN/Send CAN Data  channel=CAN_A  txlen=3  txid=hex2dec('201')  frametype=Standard(11-bit ID)  showerror=off
  wires:
  Constant/1 -> Pack Signals To CAN Data/1
  Pack Signals To CAN Data/1 -> Send CAN Data/1
  Constant1/1 -> Pack Signals To CAN Data/2
  Time interval/1 -> Pack Signals To CAN Data/3

== system VCU_TDN/Code/Asking data from the inverter/T_air ==
  Time interval : Inport
  Constant : Constant  Value=hex2dec('3d')  OutDataTypeStr=uint8
  Constant1 : Constant  Value=hex2dec('4b')  OutDataTypeStr=uint8
  Pack Signals To CAN Data : CoderSF_BSW_Libs/CAN/Pack Signals To CAN Data  Signal="{{'REG_31'  'Data1' 'Data2'},[0 8 16],[8 8 8],{'uint8'  'uint8' 'uint8'},{'Intel' 'Intel' 'Intel'}}"
  Send CAN Data : CoderSF_BSW_Libs/CAN/Send CAN Data  channel=CAN_A  txlen=3  txid=hex2dec('201')  frametype=Standard(11-bit ID)  showerror=off
  wires:
  Constant/1 -> Pack Signals To CAN Data/1
  Pack Signals To CAN Data/1 -> Send CAN Data/1
  Constant1/1 -> Pack Signals To CAN Data/2
  Time interval/1 -> Pack Signals To CAN Data/3

== system VCU_TDN/Code/Asking data from the inverter/T_motor ==
  Time interval : Inport
  Constant : Constant  Value=hex2dec('3d')  OutDataTypeStr=uint8
  Constant1 : Constant  Value=hex2dec('49')  OutDataTypeStr=uint8
  Pack Signals To CAN Data : CoderSF_BSW_Libs/CAN/Pack Signals To CAN Data  Signal="{{'REG_31'  'Data1' 'Data2'},[0 8 16],[8 8 8],{'uint8'  'uint8' 'uint8'},{'Intel' 'Intel' 'Intel'}}"
  Send CAN Data : CoderSF_BSW_Libs/CAN/Send CAN Data  channel=CAN_A  txlen=3  txid=hex2dec('201')  frametype=Standard(11-bit ID)  showerror=off
  wires:
  Constant/1 -> Pack Signals To CAN Data/1
  Pack Signals To CAN Data/1 -> Send CAN Data/1
  Constant1/1 -> Pack Signals To CAN Data/2
  Time interval/1 -> Pack Signals To CAN Data/3

== system VCU_TDN/Code/Asking data from the inverter/Vdc_bus ==
  Time interval : Inport
  Constant : Constant  Value=hex2dec('3d')  OutDataTypeStr=uint8
  Constant1 : Constant  Value=hex2dec('eb')  OutDataTypeStr=uint8
  Pack Signals To CAN Data : CoderSF_BSW_Libs/CAN/Pack Signals To CAN Data  Signal="{{'REG_31'  'Data1' 'Data2'},[0 8 16],[8 8 8],{'uint8'  'uint8' 'uint8'},{'Intel' 'Intel' 'Intel'}}"
  Send CAN Data : CoderSF_BSW_Libs/CAN/Send CAN Data  channel=CAN_A  txlen=3  txid=hex2dec('201')  frametype=Standard(11-bit ID)  showerror=off
  wires:
  Constant/1 -> Pack Signals To CAN Data/1
  Pack Signals To CAN Data/1 -> Send CAN Data/1
  Constant1/1 -> Pack Signals To CAN Data/2
  Time interval/1 -> Pack Signals To CAN Data/3

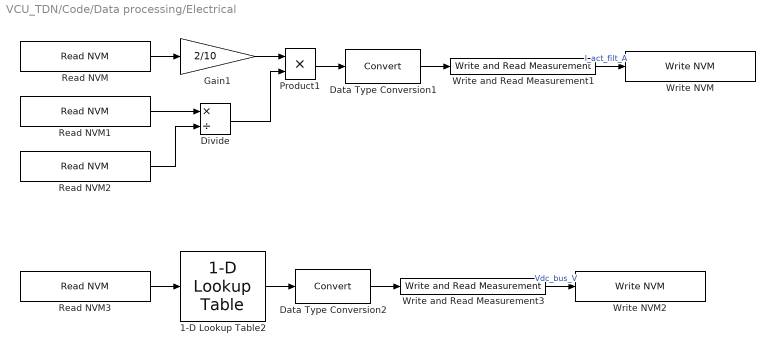
== system VCU_TDN/Code/Data processing/Electrical ==
  1-D Lookup Table2 : CoderSF_BSW_Libs/Calibration & Measurement/1-D Lookup Table  nam=Vdc_bus_V  breakpoint_type=int16  breakpoint_data=[0 748 1537 2327 3117 3906 4696 5485 6275 7065 7854 8644 9434 10223 11013 11802 12592 13382 14171 14961 15751 16540 17330 18119 18909 19699 20488 21278 22067 22857 23647 24436 25226 26016 26805 27595 28384 29174 29964 30753 31543 31751]  table_type=int16  table_data=[0 25 50 75 100 125 150 175 200 225 250 275 300 325 350 375 400 425 450 475 500 525 550 575 600 625 650 675 700 725 750 775 800 825 850 875 900 925 950 975 1000 1025]
  Data Type Conversion1 : DataTypeConversion
  Data Type Conversion2 : DataTypeConversion
  Divide : Product  Inputs=*/
  Gain1 : Gain  Gain=2/10
  Product1 : Product
  Read NVM : CoderSF_BSW_Libs/Non-volatile Memory Blocks/Read NVM  variable_name=nvmI_device  variable_type=Inherit from 'Variable definition'
  Read NVM1 : CoderSF_BSW_Libs/Non-volatile Memory Blocks/Read NVM  variable_name=nvmI_act_filt  variable_type=Inherit from 'Variable definition'
  Read NVM2 : CoderSF_BSW_Libs/Non-volatile Memory Blocks/Read NVM  variable_name=nvmI_200  variable_type=Inherit from 'Variable definition'
  Read NVM3 : CoderSF_BSW_Libs/Non-volatile Memory Blocks/Read NVM  variable_name=nvmVdc_bus  variable_type=Inherit from 'Variable definition'
  Write NVM : CoderSF_BSW_Libs/Non-volatile Memory Blocks/Write NVM  variable_name=nvmI_act_filt_A  flgDef=on  variable_value=0  variable_type=int16  variable_numD=1  unitStr=A  descStr=""  EcoCoderBlockID=N001_NVMVDEF
      settings: AttributesFormatString=value:%<variable_value> type:%<variable_type> D:%<variable_numD>
  Write NVM2 : CoderSF_BSW_Libs/Non-volatile Memory Blocks/Write NVM  variable_name=nvmVdc_bus_V  flgDef=on  variable_value=0  variable_type=int16  variable_numD=1  unitStr=V  descStr=""  EcoCoderBlockID=N001_NVMVDEF
      settings: AttributesFormatString=value:%<variable_value> type:%<variable_type> D:%<variable_numD>
  Write and Read Measurement1 : CoderSF_BSW_Libs/Calibration & Measurement/Write and Read Measurement  variable_name=I_act_filt_A  variable_value=0  variable_type=int16  numD=1  unitStr=A  descStr=""
      settings: AttributesFormatString=type:%<variable_type> Dimensions:%<numD>
  Write and Read Measurement3 : CoderSF_BSW_Libs/Calibration & Measurement/Write and Read Measurement  variable_name=Vdc_bus_V  variable_value=0  variable_type=int16  numD=1  unitStr=V  descStr=""
      settings: AttributesFormatString=type:%<variable_type> Dimensions:%<numD>
  wires:
  Product1/1 -> Data Type Conversion1/1
  Divide/1 -> Product1/2
  Read NVM2/1 -> Divide/2
  Gain1/1 -> Product1/1
  Read NVM1/1 -> Divide/1
  Data Type Conversion1/1 -> Write and Read Measurement1/1
  Read NVM/1 -> Gain1/1
  Write and Read Measurement1/1 -> Write NVM/1  "I_act_filt_A"
  1-D Lookup Table2/1 -> Data Type Conversion2/1
  Write and Read Measurement3/1 -> Write NVM2/1  "Vdc_bus_V"
  Data Type Conversion2/1 -> Write and Read Measurement3/1
  Read NVM3/1 -> 1-D Lookup Table2/1

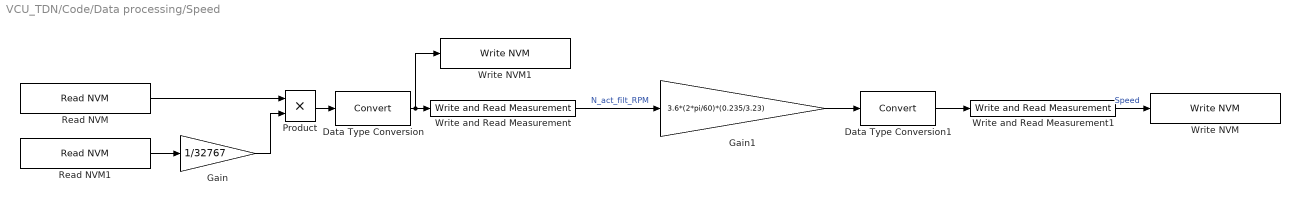
== system VCU_TDN/Code/Data processing/Speed ==
  Data Type Conversion : DataTypeConversion
  Data Type Conversion1 : DataTypeConversion
  Gain : Gain  Gain=1/32767
  Gain1 : Gain  Gain=3.6*(2*pi/60)*(0.235/3.23)
  Product : Product
  Read NVM : CoderSF_BSW_Libs/Non-volatile Memory Blocks/Read NVM  variable_name=nvmSpeedRPMmax  variable_type=Inherit from 'Variable definition'
  Read NVM1 : CoderSF_BSW_Libs/Non-volatile Memory Blocks/Read NVM  variable_name=nvmN_act_filt  variable_type=Inherit from 'Variable definition'
  Write NVM : CoderSF_BSW_Libs/Non-volatile Memory Blocks/Write NVM  variable_name=nvmSpeed  flgDef=on  variable_value=0  variable_type=int16  variable_numD=1  unitStr=km/h  descStr=""  EcoCoderBlockID=N001_NVMVDEF
      settings: AttributesFormatString=value:%<variable_value> type:%<variable_type> D:%<variable_numD>
  Write NVM1 : CoderSF_BSW_Libs/Non-volatile Memory Blocks/Write NVM  variable_name=nvmN_act_filt_RPM  flgDef=on  variable_value=0  variable_type=int16  variable_numD=1  unitStr=RPM  descStr=""  EcoCoderBlockID=N001_NVMVDEF
      settings: AttributesFormatString=value:%<variable_value> type:%<variable_type> D:%<variable_numD>
  Write and Read Measurement : CoderSF_BSW_Libs/Calibration & Measurement/Write and Read Measurement  variable_name=N_act_filt_RPM  variable_value=0  variable_type=int16  numD=1  unitStr=RPM  descStr=""
      settings: AttributesFormatString=type:%<variable_type> Dimensions:%<numD>
  Write and Read Measurement1 : CoderSF_BSW_Libs/Calibration & Measurement/Write and Read Measurement  variable_name=Speed  variable_value=0  variable_type=int16  numD=1  unitStr=km/h  descStr=""
      settings: AttributesFormatString=type:%<variable_type> Dimensions:%<numD>
  wires:
  Read NVM/1 -> Product/1
  Read NVM1/1 -> Gain/1
  Gain/1 -> Product/2
  Product/1 -> Data Type Conversion/1
  Data Type Conversion/1 -> Write NVM1/1, Write and Read Measurement/1
  Write and Read Measurement/1 -> Gain1/1  "N_act_filt_RPM"
  Gain1/1 -> Data Type Conversion1/1
  Write and Read Measurement1/1 -> Write NVM/1  "Speed"
  Data Type Conversion1/1 -> Write and Read Measurement1/1

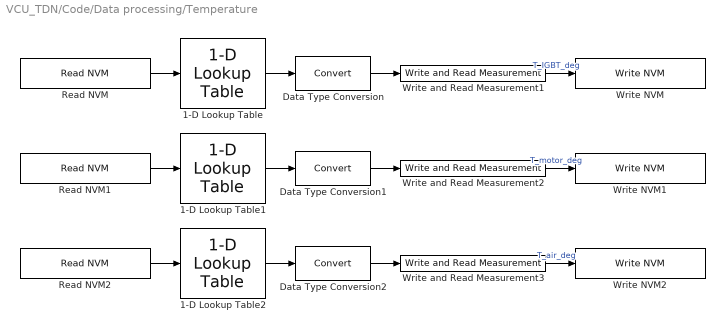
== system VCU_TDN/Code/Data processing/Temperature ==
  1-D Lookup Table : CoderSF_BSW_Libs/Calibration & Measurement/1-D Lookup Table  nam=T_IGBT_conversion  breakpoint_type=int16  breakpoint_data=[16245 16308 16387 16487 16609 16759 16938 17151 17400 17688 18017 18387 18797 19247 19733 20250 20793 21357 21933 22515 23097 23671 24232 24775 25296 25792 26261 26702 27114 27497 27851 28179 28480 28757 29011 29243 29456 29650 29827]  table_type=int16  table_data=[-35 -30 -25 -20 -15 -10 -5 0 5 10 15 20 25 30 35 40 45 50 55 60 65 70 75 80 85 90 95 100 105 110 115 120 125 130 135 140 145 150 155]
  1-D Lookup Table1 : CoderSF_BSW_Libs/Calibration & Measurement/1-D Lookup Table  nam=T_motor_conversion  breakpoint_type=int16  breakpoint_data=[7414 7687 7962 8240 8520 8802 9085 9369 9654 9939 10225 10510 10795 11080 11364 11646 11927 12207 12485 12762 13036 13308 13578 13846 14111 14373 14633 14890 15144 15391 15628 15852 16061 16251 16421 16569 16692 16789 16857]  table_type=int16  table_data=[-35 -30 -25 -20 -15 -10 -5 0 5 10 15 20 25 30 35 40 45 50 55 60 65 70 75 80 85 90 95 100 105 110 115 120 125 130 135 140 145 150 155]
  1-D Lookup Table2 : CoderSF_BSW_Libs/Calibration & Measurement/1-D Lookup Table  nam=T_air_conversion  breakpoint_type=int16  breakpoint_data=[8516 8785 9054 9322 9590 9857 10122 10386 10647 10907 11163 11418 11669 11917 12163 12404 12643 12878 13109 13337 13561 13781 13998 14210 14419 14624 14825 15022 15215]  table_type=int16  table_data=[-35 -30 -25 -20 -15 -10 -5 0 5 10 15 20 25 30 35 40 45 50 55 60 65 70 75 80 85 90 95 100 105]
  Data Type Conversion : DataTypeConversion
  Data Type Conversion1 : DataTypeConversion
  Data Type Conversion2 : DataTypeConversion
  Read NVM : CoderSF_BSW_Libs/Non-volatile Memory Blocks/Read NVM  variable_name=nvmT_IGBT  variable_type=Inherit from 'Variable definition'
  Read NVM1 : CoderSF_BSW_Libs/Non-volatile Memory Blocks/Read NVM  variable_name=nvmT_motor  variable_type=Inherit from 'Variable definition'
  Read NVM2 : CoderSF_BSW_Libs/Non-volatile Memory Blocks/Read NVM  variable_name=nvmT_air  variable_type=Inherit from 'Variable definition'
  Write NVM : CoderSF_BSW_Libs/Non-volatile Memory Blocks/Write NVM  variable_name=nvmT_IGBT_deg  flgDef=on  variable_value=0  variable_type=int16  variable_numD=1  unitStr=°C  descStr=""  EcoCoderBlockID=N001_NVMVDEF
      settings: AttributesFormatString=value:%<variable_value> type:%<variable_type> D:%<variable_numD>
  Write NVM1 : CoderSF_BSW_Libs/Non-volatile Memory Blocks/Write NVM  variable_name=nvmT_motor_deg  flgDef=on  variable_value=0  variable_type=int16  variable_numD=1  unitStr=°C  descStr=""  EcoCoderBlockID=N001_NVMVDEF
      settings: AttributesFormatString=value:%<variable_value> type:%<variable_type> D:%<variable_numD>
  Write NVM2 : CoderSF_BSW_Libs/Non-volatile Memory Blocks/Write NVM  variable_name=nvmT_air_deg  flgDef=on  variable_value=0  variable_type=int16  variable_numD=1  unitStr=°C  descStr=""  EcoCoderBlockID=N001_NVMVDEF
      settings: AttributesFormatString=value:%<variable_value> type:%<variable_type> D:%<variable_numD>
  Write and Read Measurement1 : CoderSF_BSW_Libs/Calibration & Measurement/Write and Read Measurement  variable_name=T_IGBT_deg  variable_value=0  variable_type=int16  numD=1  unitStr=°C  descStr=""
      settings: AttributesFormatString=type:%<variable_type> Dimensions:%<numD>
  Write and Read Measurement2 : CoderSF_BSW_Libs/Calibration & Measurement/Write and Read Measurement  variable_name=T_motor_deg  variable_value=0  variable_type=int16  numD=1  unitStr=°C  descStr=""
      settings: AttributesFormatString=type:%<variable_type> Dimensions:%<numD>
  Write and Read Measurement3 : CoderSF_BSW_Libs/Calibration & Measurement/Write and Read Measurement  variable_name=T_air_deg  variable_value=0  variable_type=int16  numD=1  unitStr=°C  descStr=""
      settings: AttributesFormatString=type:%<variable_type> Dimensions:%<numD>
  wires:
  Write and Read Measurement1/1 -> Write NVM/1  "T_IGBT_deg"
  Read NVM/1 -> 1-D Lookup Table/1
  Data Type Conversion/1 -> Write and Read Measurement1/1
  1-D Lookup Table/1 -> Data Type Conversion/1
  Data Type Conversion1/1 -> Write and Read Measurement2/1
  1-D Lookup Table1/1 -> Data Type Conversion1/1
  Read NVM1/1 -> 1-D Lookup Table1/1
  Write and Read Measurement2/1 -> Write NVM1/1  "T_motor_deg"
  Data Type Conversion2/1 -> Write and Read Measurement3/1
  1-D Lookup Table2/1 -> Data Type Conversion2/1
  Read NVM2/1 -> 1-D Lookup Table2/1
  Write and Read Measurement3/1 -> Write NVM2/1  "T_air_deg"
